simulink model "CNN_CA_control_six_springs"  (R2024b)
settings: Solver=VariableStepAuto  StartTime=0.0  StopTime=30  RelTol=1e-3
model workspace (MAT data in the model file):
  Camera1 = 1
undefined symbols (not defined in the file or in its folder): arm_radius, control_section_number, floor_radius, ini_arm_length, ini_spring_length, section_thickness, spring_position_scale, spring_radius, spring_stiffness, X, Y, Z
libraries: sm_lib x304, nesl_utility x156, dspindex x60, deeplib x1
(part 1 of 12)
settings Model: SimulationMode=accelerator  Creator=Fan Ye  LastModifiedBy=elija
settings SolverCC: AlgebraicLoopSolver=TrustRegion
settings OptimizationCC: ReuseModelBlockBuffer=off
settings DebuggingCC: UnconnectedInputMsg=warning  UnconnectedOutputMsg=warning  UnconnectedLineMsg=warning
settings ModelReferenceCC: EnableRefExpFcnMdlSchedulingChecks=on
settings SFSimCC: SimGenImportedTypeDefs=on  SimTargetLang=C++
settings RTWCC: GPUComputeCapability=3.5  DLArmComputeVersion=19.05
settings ExplorerConfigSet: InternalSimMechanicsExplorerSettings="<ExplorerConfiguration><canonicalview>default</canonicalview><AnimationSetting><BasePlaybackSpeed>1.0</BasePlaybackSpeed><PlaybackSpeedFactor>1.0</PlaybackSpeedFactor></AnimationSetting><TilePanel><TileInfo><Tiles Columns=\"1\" Count=\"1\" Rows=\"1\"><Column Weight=\"1\"/><Row Weight=\"1\"/><Tile Height=\"1\" Width=\"1\" X=\"0\" Y=\"0\"/></Tiles></TileInfo><SceneInfo><SceneViewer><BGColor><R>0.60000002384185791</R><G>0.60000002384185791</G><B>0.60000002384185791</B></BGColor><Camera><DoPerspective>off</DoPerspective><Position><X>0.561995715374629667</X><Y>-0.564875895152751606</Y><Z>0.957601428231976137</Z></Position><Center><X>-0.0153545538149960289</X><Y>0.0124743740368741876</Y><Z>0.380251159042350184</Z></Center><Up><X>-0.408248290463863073</X><Y>0.408248290463863073</Y><Z>0.816496580927726145</Z></Up><ViewLimDist>1</ViewLimDist><YLim>0.539098595499992506</YLim><XLim>0.631280340074036994</XLim></Camera></SceneViewer></SceneInfo></TilePanel><MechEditorPanel><Cameras/><GfxPanelCameraMap/><VideoCreator><PlaybackSpeedRatio>1.0</PlaybackSpeedRatio><FrameRate>1</FrameRate><VideoFormat>Motion JPEG AVI</VideoFormat><FrameSize>auto</FrameSize></VideoCreator></MechEditorPanel></ExplorerConfiguration>"

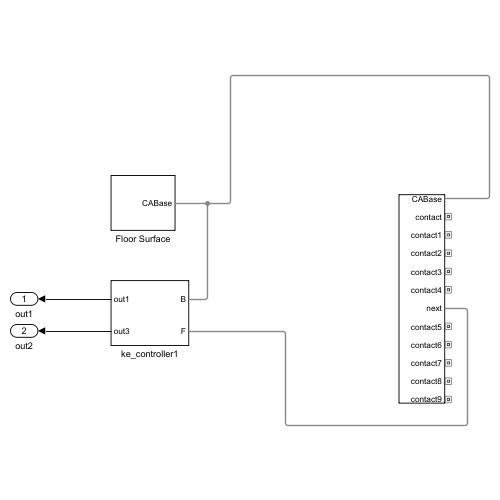
[thumbnail: Simulink's stored preview of the top-level diagram]
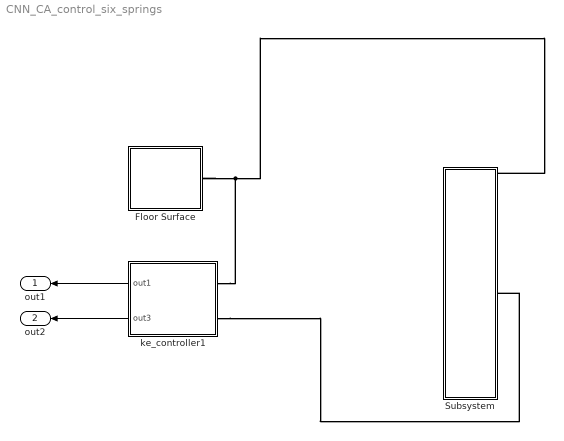
== system CNN_CA_control_six_springs ==
  Floor Surface : Subsystem  mask{length=0.5, width=0.5, floor_radius=floor_radius, floor_thickness=section_thickness, floor_density=1000}
      mask prompts: length "grid length [m]"; width "grid width [m]"; floor_radius "floor radius [m]"; floor_thickness "floor thickness [m]"; floor_density "floor density [kg/m^3]"
  Subsystem : Subsystem  mask{damping=10000}
  ke_controller1 : Subsystem  mask{time=1/10}
      settings: PortSchema="{\"entries\":[{\"content\":{\"sides\":[{\"content\":{\"connectorIds\":[\"Out1\",\"Out2\"]},\"type\":\"ConnectorPlacement.EquallySpacedRectSide\",\"uuid\":\"040155ee-60b1-421c-8328-c25461da302b\"},{\"content\":{\"connectorIds\":[\"RConn1\",\"RConn2\"],\"side\":\"RIGHT\"},\"type\":\"ConnectorPlacement.EquallySpacedRectSide\",\"uuid\":\"fd708fec-fd39-4a33-8156-5c69a86363e4\"},{\"content\":{\"connectorIds\":[],\"side\":\"TOP\"},\"type\":\"ConnectorPlacement.EquallySpacedRectSide\",\"uuid\":\"3eab7f87-5dcc-46aa-aa6d-ebff8fc02a1f\"},{\"content\":{\"connectorIds\":[],\"side\":\"HIDDEN\"},\"type\":\"ConnectorPlacement.EquallySpacedRectSide\",\"uuid\":\"eabd9a25-303c-4f3d-a71b-72a20e95be15\"}]},\"type\":\"ConnectorPlacement.EquallySpacedConnector\",\"uuid\":\"7f057b11-92ee-4c15-b9f6-e9a247ee9eef\"}],\"packageUris\":[\"http://schema.mathworks.com/mf0/Connector/R2020b\"],\"version\":\"1.0\"}"
  out1 : Outport
  out2 : Outport  Port=2
  wires:
  ke_controller1/1(out1) -> out1/1
  ke_controller1/2(out3) -> out2/1
  connections:
  Floor Surface/RConn1 -- ke_controller1/RConn1 -- Subsystem/RConn1
  ke_controller1/RConn2 -- Subsystem/RConn7

== system CNN_CA_control_six_springs/Floor Surface ==
  Floor : Subsystem  AncestorBlock=RP_Simulator_Components/Obstacle Arena/Floor
      settings: LibrarySourceBlock=RP_Simulator_Components/Obstacle Arena/Floor
  Mechanism Configuration1 : sm_lib/Utilities/Mechanism Configuration  UniformGravity=Constant  GravityVector=[0 0 9.80665]  GravityVectorUnits=m/s^2  LinearizationDelta=0.001  JointModeTransitionNonlinearIterations=2
  Solver Configuration1 : nesl_utility/Solver Configuration  PhysicalDomain=network_engine_domain  SubClassName=solver  LeftPortType=input  RightPortType=generic  Tones=[]  Harmonics=[]  SimulateNoise=off  Profile=off  UseLocalSampling=off  EnableSwitchedLinearOptims=on  FrequencyDomain=off  UseCCode=off  RelTol=0.001  AbsTol=1e-06  MinStep=1e-09  ToWorkspace=off  RevertToSquareIcSolve=off  NumHomotopyIterations=100  PhasorMode=off  PhasorModeNumHarmonics=1  ConsistencySolver=NEWTON_FTOL  IndexReductionMethod=DerivativeReplacement  DoDC=off  ResidualTolerance=1e-09  ConsistencyTolSource=GLOBAL  ConsistencyAbsTol=0.001  ConsistencyRelTol=0.001  ConsistencyTolFactor=0.001  UseLocalSolver=off  LocalSolverChoice=NE_BACKWARD_EULER_ADVANCER  ResolveIndetEquations=on  FunctionEvalNumThread=1  LocalSolverSampleTime=0.0002  DoFixedCost=off  MaxNonlinIter=10  MaxModeIter=2  ComputeImpulses=off  ImpulseIterations=2  LinearAlgebra=Sparse  LinearAlgebraNumThread=0  EquationFormulation=NE_TIME_EF  DelaysMemoryBudget=1024  AutomaticFiltering=off  FilteringTimeConstant=0.001  PartitionStorageMethod=AS_NEEDED  PartitionMemoryBudget=1024  PartitionMethod=FAST  MultibodyUseLocalSolver=off  MultibodyLocalSolverChoice=ODE1  MultibodyLocalSolverSampleTime=0.001
  World Frame1 : sm_lib/Frames and Transforms/World Frame
  CABase : PMIOPort  Side=Right
  connections:
  Floor/RConn1 -- CABase/RConn1 -- Mechanism Configuration1/RConn1 -- World Frame1/RConn1 -- Solver Configuration1/RConn1

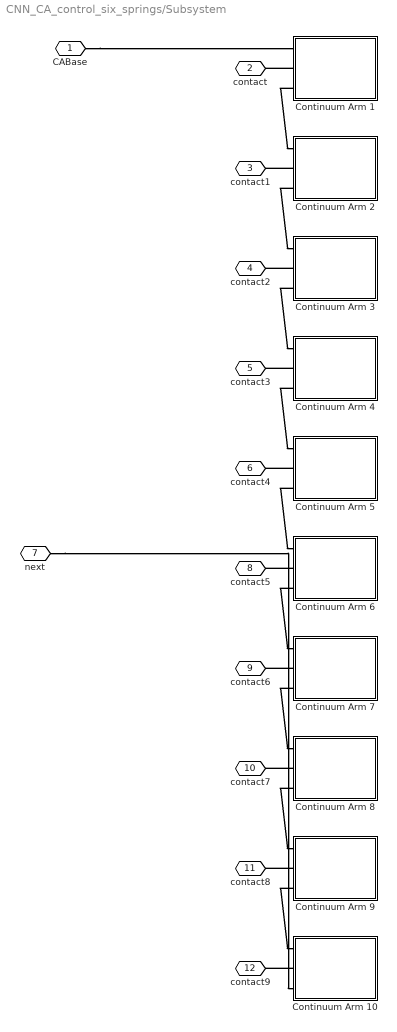
== system CNN_CA_control_six_springs/Subsystem ==
  Continuum Arm 1 : Subsystem  mask{arm_radius=arm_radius(1), arm_radius_previus=floor_radius, arm_thickness=section_thickness, arm_mass=0.00001, spring_radius=spring_radius(1), spring_mass=0.00001, ini_arm_length=ini_arm_length(1), column_number=control_section_number(1), spring_position_scale_1=spring_position_scale(1,1), spring_stiffness_1=spring_stiffness(1,1), damping_coefficient_1=damping, ini_spring_length_1=ini_spring_length(1,1), spring_position_scale_2=spring_position_scale(1,2), spring_stiffness_2=spring_stiffness(1,2), damping_coefficient_2=damping, ini_spring_length_2=ini_spring_length(1,2), spring_position_scale_3=spring_position_scale(1,3), spring_stiffness_3=spring_stiffness(1,3), damping_coefficient_3=damping, ini_spring_length_3=ini_spring_length(1,3)}
      mask prompts: arm_radius "arm radius [m]"; arm_radius_previus "arm radius previus [m]"; arm_thickness "arm thickness [m]"; arm_mass "arm mass [kg]"; spring_radius "spring radius [m]"; spring_mass "spring mass [kg]"; ini_arm_length "ini arm length [m]"; column_number "control section number"; spring_position_scale_1 "spring position scale"; spring_stiffness_1 "spring stiffness [N/m]"; damping_coefficient_1 "damping coefficient [N/(m/s)]"; ini_spring_length_1 "ini spring length [m]"; spring_position_scale_2 "spring position scale"; spring_stiffness_2 "spring stiffness [N/m]"; damping_coefficient_2 "damping coefficient [N/(m/s)]"; ini_spring_length_2 "ini spring length [m]"; spring_position_scale_3 "spring position scale"; spring_stiffness_3 "spring stiffness [N/m]"; damping_coefficient_3 "damping coefficient [N/(m/s)]"; ini_spring_length_3 "ini spring length [m]"
      mask DialogControl spring1 Prompt: spring1
      mask DialogControl spring2 Prompt: spring2
      mask DialogControl spring3 Prompt: spring3
  Continuum Arm 10 : Subsystem  mask{arm_radius=arm_radius(10), arm_radius_previus=arm_radius(9), arm_thickness=section_thickness, arm_mass=0.00001, spring_radius=spring_radius(10), spring_mass=0.00001, ini_arm_length=ini_arm_length(10), column_number=control_section_number(10), spring_position_scale_1=spring_position_scale(10,1), spring_stiffness_1=spring_stiffness(10,1), damping_coefficient_1=damping, ini_spring_length_1=ini_spring_length(10,1), spring_position_scale_2=spring_position_scale(10,2), spring_stiffness_2=spring_stiffness(10,2), damping_coefficient_2=damping, ini_spring_length_2=ini_spring_length(10,2), spring_position_scale_3=spring_position_scale(10,3), spring_stiffness_3=spring_stiffness(10,3), damping_coefficient_3=damping, ini_spring_length_3=ini_spring_length(10,3)}
      mask prompts: arm_radius "arm radius [m]"; arm_radius_previus "arm radius previus [m]"; arm_thickness "arm thickness [m]"; arm_mass "arm mass [kg]"; spring_radius "spring radius [m]"; spring_mass "spring mass [kg]"; ini_arm_length "ini arm length [m]"; column_number "control section number"; spring_position_scale_1 "spring position scale"; spring_stiffness_1 "spring stiffness [N/m]"; damping_coefficient_1 "damping coefficient [N/(m/s)]"; ini_spring_length_1 "ini spring length [m]"; spring_position_scale_2 "spring position scale"; spring_stiffness_2 "spring stiffness [N/m]"; damping_coefficient_2 "damping coefficient [N/(m/s)]"; ini_spring_length_2 "ini spring length [m]"; spring_position_scale_3 "spring position scale"; spring_stiffness_3 "spring stiffness [N/m]"; damping_coefficient_3 "damping coefficient [N/(m/s)]"; ini_spring_length_3 "ini spring length [m]"
      mask DialogControl spring1 Prompt: spring1
      mask DialogControl spring2 Prompt: spring2
      mask DialogControl spring3 Prompt: spring3
  Continuum Arm 2 : Subsystem  mask{arm_radius=arm_radius(2), arm_radius_previus=arm_radius(1), arm_thickness=section_thickness, arm_mass=0.00001, spring_radius=spring_radius(2), spring_mass=0.00001, ini_arm_length=ini_arm_length(2), column_number=control_section_number(2), spring_position_scale_1=spring_position_scale(2,1), spring_stiffness_1=spring_stiffness(2,1), damping_coefficient_1=damping, ini_spring_length_1=ini_spring_length(2,1), spring_position_scale_2=spring_position_scale(2,2), spring_stiffness_2=spring_stiffness(2,2), damping_coefficient_2=damping, ini_spring_length_2=ini_spring_length(2,2), spring_position_scale_3=spring_position_scale(2,3), spring_stiffness_3=spring_stiffness(2,3), damping_coefficient_3=damping, ini_spring_length_3=ini_spring_length(2,3)}
      mask prompts: arm_radius "arm radius [m]"; arm_radius_previus "arm radius previus [m]"; arm_thickness "arm thickness [m]"; arm_mass "arm mass [kg]"; spring_radius "spring radius [m]"; spring_mass "spring mass [kg]"; ini_arm_length "ini arm length [m]"; column_number "control section number"; spring_position_scale_1 "spring position scale"; spring_stiffness_1 "spring stiffness [N/m]"; damping_coefficient_1 "damping coefficient [N/(m/s)]"; ini_spring_length_1 "ini spring length [m]"; spring_position_scale_2 "spring position scale"; spring_stiffness_2 "spring stiffness [N/m]"; damping_coefficient_2 "damping coefficient [N/(m/s)]"; ini_spring_length_2 "ini spring length [m]"; spring_position_scale_3 "spring position scale"; spring_stiffness_3 "spring stiffness [N/m]"; damping_coefficient_3 "damping coefficient [N/(m/s)]"; ini_spring_length_3 "ini spring length [m]"
      mask DialogControl spring1 Prompt: spring1
      mask DialogControl spring2 Prompt: spring2
      mask DialogControl spring3 Prompt: spring3
  Continuum Arm 3 : Subsystem  mask{arm_radius=arm_radius(3), arm_radius_previus=arm_radius(2), arm_thickness=section_thickness, arm_mass=0.00001, spring_radius=spring_radius(3), spring_mass=0.00001, ini_arm_length=ini_arm_length(3), column_number=control_section_number(3), spring_position_scale_1=spring_position_scale(3,1), spring_stiffness_1=spring_stiffness(3,1), damping_coefficient_1=damping, ini_spring_length_1=ini_spring_length(3,1), spring_position_scale_2=spring_position_scale(3,2), spring_stiffness_2=spring_stiffness(3,2), damping_coefficient_2=damping, ini_spring_length_2=ini_spring_length(3,2), spring_position_scale_3=spring_position_scale(3,3), spring_stiffness_3=spring_stiffness(3,3), damping_coefficient_3=damping, ini_spring_length_3=ini_spring_length(3,3)}
      mask prompts: arm_radius "arm radius [m]"; arm_radius_previus "arm radius previus [m]"; arm_thickness "arm thickness [m]"; arm_mass "arm mass [kg]"; spring_radius "spring radius [m]"; spring_mass "spring mass [kg]"; ini_arm_length "ini arm length [m]"; column_number "control section number"; spring_position_scale_1 "spring position scale"; spring_stiffness_1 "spring stiffness [N/m]"; damping_coefficient_1 "damping coefficient [N/(m/s)]"; ini_spring_length_1 "ini spring length [m]"; spring_position_scale_2 "spring position scale"; spring_stiffness_2 "spring stiffness [N/m]"; damping_coefficient_2 "damping coefficient [N/(m/s)]"; ini_spring_length_2 "ini spring length [m]"; spring_position_scale_3 "spring position scale"; spring_stiffness_3 "spring stiffness [N/m]"; damping_coefficient_3 "damping coefficient [N/(m/s)]"; ini_spring_length_3 "ini spring length [m]"
      mask DialogControl spring1 Prompt: spring1
      mask DialogControl spring2 Prompt: spring2
      mask DialogControl spring3 Prompt: spring3
  Continuum Arm 4 : Subsystem  mask{arm_radius=arm_radius(4), arm_radius_previus=arm_radius(3), arm_thickness=section_thickness, arm_mass=0.00001, spring_radius=spring_radius(4), spring_mass=0.00001, ini_arm_length=ini_arm_length(4), column_number=control_section_number(4), spring_position_scale_1=spring_position_scale(4,1), spring_stiffness_1=spring_stiffness(4,1), damping_coefficient_1=damping, ini_spring_length_1=ini_spring_length(4,1), spring_position_scale_2=spring_position_scale(4,2), spring_stiffness_2=spring_stiffness(4,2), damping_coefficient_2=damping, ini_spring_length_2=ini_spring_length(4,2), spring_position_scale_3=spring_position_scale(4,3), spring_stiffness_3=spring_stiffness(4,3), damping_coefficient_3=damping, ini_spring_length_3=ini_spring_length(4,3)}
      mask prompts: arm_radius "arm radius [m]"; arm_radius_previus "arm radius previus [m]"; arm_thickness "arm thickness [m]"; arm_mass "arm mass [kg]"; spring_radius "spring radius [m]"; spring_mass "spring mass [kg]"; ini_arm_length "ini arm length [m]"; column_number "control section number"; spring_position_scale_1 "spring position scale"; spring_stiffness_1 "spring stiffness [N/m]"; damping_coefficient_1 "damping coefficient [N/(m/s)]"; ini_spring_length_1 "ini spring length [m]"; spring_position_scale_2 "spring position scale"; spring_stiffness_2 "spring stiffness [N/m]"; damping_coefficient_2 "damping coefficient [N/(m/s)]"; ini_spring_length_2 "ini spring length [m]"; spring_position_scale_3 "spring position scale"; spring_stiffness_3 "spring stiffness [N/m]"; damping_coefficient_3 "damping coefficient [N/(m/s)]"; ini_spring_length_3 "ini spring length [m]"
      mask DialogControl spring1 Prompt: spring1
      mask DialogControl spring2 Prompt: spring2
      mask DialogControl spring3 Prompt: spring3
  Continuum Arm 5 : Subsystem  mask{arm_radius=arm_radius(5), arm_radius_previus=arm_radius(4), arm_thickness=section_thickness, arm_mass=0.00001, spring_radius=spring_radius(5), spring_mass=0.00001, ini_arm_length=ini_arm_length(5), column_number=control_section_number(5), spring_position_scale_1=spring_position_scale(5,1), spring_stiffness_1=spring_stiffness(5,1), damping_coefficient_1=damping, ini_spring_length_1=ini_spring_length(5,1), spring_position_scale_2=spring_position_scale(5,2), spring_stiffness_2=spring_stiffness(5,2), damping_coefficient_2=damping, ini_spring_length_2=ini_spring_length(5,2), spring_position_scale_3=spring_position_scale(5,3), spring_stiffness_3=spring_stiffness(5,3), damping_coefficient_3=damping, ini_spring_length_3=ini_spring_length(5,3)}
      mask prompts: arm_radius "arm radius [m]"; arm_radius_previus "arm radius previus [m]"; arm_thickness "arm thickness [m]"; arm_mass "arm mass [kg]"; spring_radius "spring radius [m]"; spring_mass "spring mass [kg]"; ini_arm_length "ini arm length [m]"; column_number "control section number"; spring_position_scale_1 "spring position scale"; spring_stiffness_1 "spring stiffness [N/m]"; damping_coefficient_1 "damping coefficient [N/(m/s)]"; ini_spring_length_1 "ini spring length [m]"; spring_position_scale_2 "spring position scale"; spring_stiffness_2 "spring stiffness [N/m]"; damping_coefficient_2 "damping coefficient [N/(m/s)]"; ini_spring_length_2 "ini spring length [m]"; spring_position_scale_3 "spring position scale"; spring_stiffness_3 "spring stiffness [N/m]"; damping_coefficient_3 "damping coefficient [N/(m/s)]"; ini_spring_length_3 "ini spring length [m]"
      mask DialogControl spring1 Prompt: spring1
      mask DialogControl spring2 Prompt: spring2
      mask DialogControl spring3 Prompt: spring3
  Continuum Arm 6 : Subsystem  mask{arm_radius=arm_radius(6), arm_radius_previus=arm_radius(5), arm_thickness=section_thickness, arm_mass=0.00001, spring_radius=spring_radius(6), spring_mass=0.00001, ini_arm_length=ini_arm_length(6), column_number=control_section_number(6), spring_position_scale_1=spring_position_scale(6,1), spring_stiffness_1=spring_stiffness(6,1), damping_coefficient_1=damping, ini_spring_length_1=ini_spring_length(6,1), spring_position_scale_2=spring_position_scale(6,2), spring_stiffness_2=spring_stiffness(6,2), damping_coefficient_2=damping, ini_spring_length_2=ini_spring_length(6,2), spring_position_scale_3=spring_position_scale(6,3), spring_stiffness_3=spring_stiffness(6,3), damping_coefficient_3=damping, ini_spring_length_3=ini_spring_length(6,3)}
      mask prompts: arm_radius "arm radius [m]"; arm_radius_previus "arm radius previus [m]"; arm_thickness "arm thickness [m]"; arm_mass "arm mass [kg]"; spring_radius "spring radius [m]"; spring_mass "spring mass [kg]"; ini_arm_length "ini arm length [m]"; column_number "control section number"; spring_position_scale_1 "spring position scale"; spring_stiffness_1 "spring stiffness [N/m]"; damping_coefficient_1 "damping coefficient [N/(m/s)]"; ini_spring_length_1 "ini spring length [m]"; spring_position_scale_2 "spring position scale"; spring_stiffness_2 "spring stiffness [N/m]"; damping_coefficient_2 "damping coefficient [N/(m/s)]"; ini_spring_length_2 "ini spring length [m]"; spring_position_scale_3 "spring position scale"; spring_stiffness_3 "spring stiffness [N/m]"; damping_coefficient_3 "damping coefficient [N/(m/s)]"; ini_spring_length_3 "ini spring length [m]"
      mask DialogControl spring1 Prompt: spring1
      mask DialogControl spring2 Prompt: spring2
      mask DialogControl spring3 Prompt: spring3
  Continuum Arm 7 : Subsystem  mask{arm_radius=arm_radius(7), arm_radius_previus=arm_radius(6), arm_thickness=section_thickness, arm_mass=0.00001, spring_radius=spring_radius(7), spring_mass=0.00001, ini_arm_length=ini_arm_length(7), column_number=control_section_number(7), spring_position_scale_1=spring_position_scale(7,1), spring_stiffness_1=spring_stiffness(7,1), damping_coefficient_1=damping, ini_spring_length_1=ini_spring_length(7,1), spring_position_scale_2=spring_position_scale(7,2), spring_stiffness_2=spring_stiffness(7,2), damping_coefficient_2=damping, ini_spring_length_2=ini_spring_length(7,2), spring_position_scale_3=spring_position_scale(7,3), spring_stiffness_3=spring_stiffness(7,3), damping_coefficient_3=damping, ini_spring_length_3=ini_spring_length(7,3)}
      mask prompts: arm_radius "arm radius [m]"; arm_radius_previus "arm radius previus [m]"; arm_thickness "arm thickness [m]"; arm_mass "arm mass [kg]"; spring_radius "spring radius [m]"; spring_mass "spring mass [kg]"; ini_arm_length "ini arm length [m]"; column_number "control section number"; spring_position_scale_1 "spring position scale"; spring_stiffness_1 "spring stiffness [N/m]"; damping_coefficient_1 "damping coefficient [N/(m/s)]"; ini_spring_length_1 "ini spring length [m]"; spring_position_scale_2 "spring position scale"; spring_stiffness_2 "spring stiffness [N/m]"; damping_coefficient_2 "damping coefficient [N/(m/s)]"; ini_spring_length_2 "ini spring length [m]"; spring_position_scale_3 "spring position scale"; spring_stiffness_3 "spring stiffness [N/m]"; damping_coefficient_3 "damping coefficient [N/(m/s)]"; ini_spring_length_3 "ini spring length [m]"
      mask DialogControl spring1 Prompt: spring1
      mask DialogControl spring2 Prompt: spring2
      mask DialogControl spring3 Prompt: spring3
  Continuum Arm 8 : Subsystem  mask{arm_radius=arm_radius(8), arm_radius_previus=arm_radius(7), arm_thickness=section_thickness, arm_mass=0.00001, spring_radius=spring_radius(8), spring_mass=0.00001, ini_arm_length=ini_arm_length(8), column_number=control_section_number(8), spring_position_scale_1=spring_position_scale(8,1), spring_stiffness_1=spring_stiffness(8,1), damping_coefficient_1=damping, ini_spring_length_1=ini_spring_length(8,1), spring_position_scale_2=spring_position_scale(8,2), spring_stiffness_2=spring_stiffness(8,2), damping_coefficient_2=damping, ini_spring_length_2=ini_spring_length(8,2), spring_position_scale_3=spring_position_scale(8,3), spring_stiffness_3=spring_stiffness(8,3), damping_coefficient_3=damping, ini_spring_length_3=ini_spring_length(8,3)}
      mask prompts: arm_radius "arm radius [m]"; arm_radius_previus "arm radius previus [m]"; arm_thickness "arm thickness [m]"; arm_mass "arm mass [kg]"; spring_radius "spring radius [m]"; spring_mass "spring mass [kg]"; ini_arm_length "ini arm length [m]"; column_number "control section number"; spring_position_scale_1 "spring position scale"; spring_stiffness_1 "spring stiffness [N/m]"; damping_coefficient_1 "damping coefficient [N/(m/s)]"; ini_spring_length_1 "ini spring length [m]"; spring_position_scale_2 "spring position scale"; spring_stiffness_2 "spring stiffness [N/m]"; damping_coefficient_2 "damping coefficient [N/(m/s)]"; ini_spring_length_2 "ini spring length [m]"; spring_position_scale_3 "spring position scale"; spring_stiffness_3 "spring stiffness [N/m]"; damping_coefficient_3 "damping coefficient [N/(m/s)]"; ini_spring_length_3 "ini spring length [m]"
      mask DialogControl spring1 Prompt: spring1
      mask DialogControl spring2 Prompt: spring2
      mask DialogControl spring3 Prompt: spring3
  Continuum Arm 9 : Subsystem  mask{arm_radius=arm_radius(9), arm_radius_previus=arm_radius(8), arm_thickness=section_thickness, arm_mass=0.00001, spring_radius=spring_radius(9), spring_mass=0.00001, ini_arm_length=ini_arm_length(9), column_number=control_section_number(9), spring_position_scale_1=spring_position_scale(9,1), spring_stiffness_1=spring_stiffness(9,1), damping_coefficient_1=damping, ini_spring_length_1=ini_spring_length(9,1), spring_position_scale_2=spring_position_scale(9,2), spring_stiffness_2=spring_stiffness(9,2), damping_coefficient_2=damping, ini_spring_length_2=ini_spring_length(9,2), spring_position_scale_3=spring_position_scale(9,3), spring_stiffness_3=spring_stiffness(9,3), damping_coefficient_3=damping, ini_spring_length_3=ini_spring_length(9,3)}
      mask prompts: arm_radius "arm radius [m]"; arm_radius_previus "arm radius previus [m]"; arm_thickness "arm thickness [m]"; arm_mass "arm mass [kg]"; spring_radius "spring radius [m]"; spring_mass "spring mass [kg]"; ini_arm_length "ini arm length [m]"; column_number "control section number"; spring_position_scale_1 "spring position scale"; spring_stiffness_1 "spring stiffness [N/m]"; damping_coefficient_1 "damping coefficient [N/(m/s)]"; ini_spring_length_1 "ini spring length [m]"; spring_position_scale_2 "spring position scale"; spring_stiffness_2 "spring stiffness [N/m]"; damping_coefficient_2 "damping coefficient [N/(m/s)]"; ini_spring_length_2 "ini spring length [m]"; spring_position_scale_3 "spring position scale"; spring_stiffness_3 "spring stiffness [N/m]"; damping_coefficient_3 "damping coefficient [N/(m/s)]"; ini_spring_length_3 "ini spring length [m]"
      mask DialogControl spring1 Prompt: spring1
      mask DialogControl spring2 Prompt: spring2
      mask DialogControl spring3 Prompt: spring3
  CABase : PMIOPort  Side=Right
  contact : PMIOPort  Port=2  Side=Right
  contact1 : PMIOPort  Port=3  Side=Right
  contact2 : PMIOPort  Port=4  Side=Right
  contact3 : PMIOPort  Port=5  Side=Right
  contact4 : PMIOPort  Port=6  Side=Right
  next : PMIOPort  Port=7  Side=Right
  contact5 : PMIOPort  Port=8  Side=Right
  contact6 : PMIOPort  Port=9  Side=Right
  contact7 : PMIOPort  Port=10  Side=Right
  contact8 : PMIOPort  Port=11  Side=Right
  contact9 : PMIOPort  Port=12  Side=Right
  connections:
  Continuum Arm 1/RConn3 -- Continuum Arm 2/RConn1
  Continuum Arm 3/RConn3 -- Continuum Arm 4/RConn1
  Continuum Arm 7/RConn3 -- Continuum Arm 8/RConn1
  Continuum Arm 2/RConn2 -- contact1/RConn1
  Continuum Arm 8/RConn3 -- Continuum Arm 9/RConn1
  Continuum Arm 2/RConn3 -- Continuum Arm 3/RConn1
  Continuum Arm 6/RConn3 -- Continuum Arm 7/RConn1
  Continuum Arm 3/RConn2 -- contact2/RConn1
  Continuum Arm 5/RConn3 -- Continuum Arm 6/RConn1
  Continuum Arm 9/RConn3 -- Continuum Arm 10/RConn1
  Continuum Arm 4/RConn3 -- Continuum Arm 5/RConn1
  next/RConn1 -- Continuum Arm 10/RConn3
  CABase/RConn1 -- Continuum Arm 1/RConn1
  Continuum Arm 5/RConn2 -- contact4/RConn1
  Continuum Arm 1/RConn2 -- contact/RConn1
  Continuum Arm 9/RConn2 -- contact8/RConn1
  Continuum Arm 10/RConn2 -- contact9/RConn1
  Continuum Arm 7/RConn2 -- contact6/RConn1
  Continuum Arm 8/RConn2 -- contact7/RConn1
  Continuum Arm 4/RConn2 -- contact3/RConn1
  Continuum Arm 6/RConn2 -- contact5/RConn1

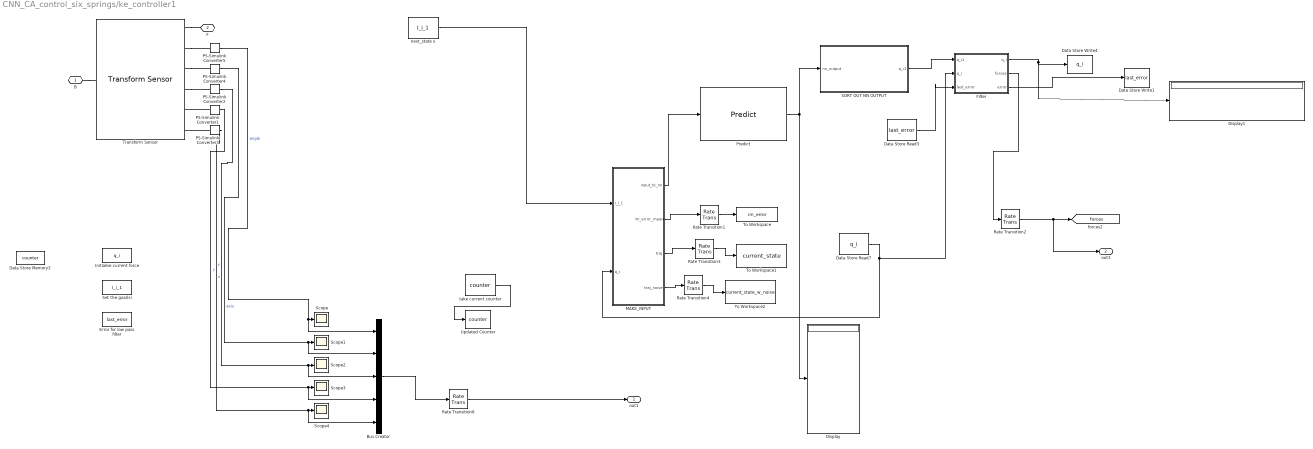
== system CNN_CA_control_six_springs/ke_controller1 ==
  Bus Creator : BusCreator  Inputs=5
  Data Store Memory3 : DataStoreMemory  DataStoreName=counter  WriteAfterWriteMsg=warning  InitialValue=counter  ShowAdditionalParam=off
  Data Store Read3 : DataStoreRead  DataStoreName=last_error  IndexOptions=Index vector (dialog)  Indices=1  OutputSizes=1
  Data Store Read7 : DataStoreRead  DataStoreName=q_i  IndexOptions=Index vector (dialog)  Indices=1  OutputSizes=1
  Data Store Write1 : DataStoreWrite  DataStoreName=last_error  IndexOptions=Index vector (dialog)  Indices=1  OutputSizes=1
  Data Store Write4 : DataStoreWrite  DataStoreName=q_i  IndexOptions=Index vector (dialog)  Indices=1  OutputSizes=1
  Display : Display
  Display1 : Display
  Error for low pass filter : DataStoreMemory  DataStoreName=last_error  WriteAfterWriteMsg=warning  InitialValue=last_error  ShowAdditionalParam=off
  Filter : MATLAB Function  TreatAsAtomicUnit=on  SystemSampleTime=time
  Initialise current force : DataStoreMemory  DataStoreName=q_i  WriteAfterWriteMsg=warning  InitialValue=q_i  ShowAdditionalParam=off
  MAKE_INPUT : MATLAB Function  TreatAsAtomicUnit=on  SystemSampleTime=time
  PS-Simulink Converter{1..5} (5 alike) : nesl_utility/PS-Simulink Converter  PhysicalDomain=network_engine_domain  SubClassName=ps_output  LeftPortType=input  RightPortType=output  PseudoPeriodic=off  Frequencies=[]  VectorFormat=1-D array  Unit=1  AffineConversion=off
  Predict : deeplib/Predict  Network=Network from MAT-file  NetworkFunction=squeezenet  NetworkFilePath=.\variable_net6_best.mat  MiniBatchSize=1  InputDataFormats={'',''}  Predictions=on  Activations={}  ForceInterpretedSim=off  EnableDLNetwork=on  LastKnownNetworkFilePath=''  LastKnownNetworkTimeStamp=''
  Rate Transition{1..4,8} (5 alike) : RateTransition  OutPortSampleTime=time
  SORT OUT NN OUTPUT : MATLAB Function  TreatAsAtomicUnit=on  SystemSampleTime=0.1
  Scope{,1..4} (5 alike) : Scope
  Set the goal(s) : DataStoreMemory  DataStoreName=I_i_1  WriteAfterWriteMsg=warning  InitialValue=I_i_1  ShowAdditionalParam=off
  To Workspace : ToWorkspace  VariableName=im_error  SaveFormat=Timeseries  SampleTime=-1
  To Workspace1 : ToWorkspace  VariableName=current_state  SaveFormat=Timeseries  SampleTime=-1
  To Workspace2 : ToWorkspace  VariableName=current_state_w_noise  SaveFormat=Timeseries  SampleTime=-1
  Transform Sensor : sm_lib/Frames and Transforms/Transform Sensor  MeasurementFrame=World  RotationSequence=XYX  SenseAngle=on  SenseAxis=on  SenseQ=off  SenseR=off  SenseRotationSequence=off  SenseOmegaX=off  SenseOmegaY=off  SenseOmegaZ=off  SenseOmega=off  SenseQDot=off  SenseRDot=off  SenseRotationSequenceDot=off  SenseAlphaX=off  SenseAlphaY=off  SenseAlphaZ=off  SenseAlpha=off  SenseQDDot=off  SenseRDDot=off  SenseX=on  SenseY=on  SenseZ=on  SenseXYZ=off  SenseRad=off  SenseAzim=off  SenseDist=off  SenseInc=off  SenseXDot=off  SenseYDot=off  SenseZDot=off  SenseXYZDot=off  SenseRadDot=off  SenseAzimDot=off  SenseDistDot=off  SenseIncDot=off  SenseXDDot=off  SenseYDDot=off  SenseZDDot=off  SenseXYZDDot=off  SenseRadDDot=off  SenseAzimDDot=off  SenseDistDDot=off  SenseIncDDot=off
  Updated Counter : DataStoreWrite  DataStoreName=counter  IndexOptions=Index vector (dialog)  Indices=1  OutputSizes=1
  next_state x : DataStoreRead  DataStoreName=I_i_1  IndexOptions=Index vector (dialog)  Indices=1  OutputSizes=1
  take current counter : DataStoreRead  DataStoreName=counter  IndexOptions=Index vector (dialog)  Indices=1  OutputSizes=1
  B : PMIOPort  Side=Right
  F : PMIOPort  Port=2  Side=Right
  out1 : Outport
  out3 : Outport  Port=2
  tag scope: forces=global
  wires:
  PS-Simulink Converter3/1 -> Bus Creator/5, Scope4/1  "z"
  PS-Simulink Converter1/1 -> Bus Creator/4, Scope3/1  "y"
  PS-Simulink Converter2/1 -> Bus Creator/3, Scope2/1  "x"
  PS-Simulink Converter4/1 -> Bus Creator/2, Scope1/1  "axis"
  PS-Simulink Converter5/1 -> Bus Creator/1, Scope/1  "angle"
  Bus Creator/1 -> Rate Transition8/1
  Rate Transition8/1 -> out1/1
  take current counter/1 -> Updated Counter/1
  MAKE_INPUT/1(input_to_nn) -> Predict/1
  Predict/1 -> Display/1, SORT OUT NN OUTPUT/1(nn_output)
  SORT OUT NN OUTPUT/1(q_i1) -> Filter/1(q_i1)
  next_state x/1 -> MAKE_INPUT/1(I_i_1)
  Data Store Read7/1 -> Filter/2("q_i "), MAKE_INPUT/2(q_i)
  Filter/1(q_i) -> Display1/1, Data Store Write4/1
  Rate Transition2/1 -> out3/1, [forces]
  Filter/2(forces) -> Rate Transition2/1
  Data Store Read3/1 -> Filter/3(last_error)
  Filter/3(error) -> Data Store Write1/1
  MAKE_INPUT/2(im_error_mean) -> Rate Transition1/1
  Rate Transition1/1 -> To Workspace/1
  MAKE_INPUT/3(traj) -> Rate Transition3/1
  Rate Transition3/1 -> To Workspace1/1
  Rate Transition4/1 -> To Workspace2/1
  MAKE_INPUT/4(traj_noise) -> Rate Transition4/1
  connections:
  PS-Simulink Converter3/LConn1 -- Transform Sensor/RConn6
  PS-Simulink Converter1/LConn1 -- Transform Sensor/RConn5
  Transform Sensor/RConn4 -- PS-Simulink Converter2/LConn1
  Transform Sensor/RConn3 -- PS-Simulink Converter4/LConn1
  Transform Sensor/RConn2 -- PS-Simulink Converter5/LConn1
  B/RConn1 -- Transform Sensor/LConn1
  Transform Sensor/RConn1 -- F/RConn1

== system CNN_CA_control_six_springs/Floor Surface/Floor ==
  Floor : sm_lib/Body Elements/Cylindrical Solid  CylinderRadius=floor_radius  CylinderRadiusUnits=m  CylinderLength=floor_thickness  CylinderLengthUnits=m  ExportEntireGeometry=on  InertiaType=CalculateFromGeometry  BasedOnType=Density  Density=floor_density  DensityUnits=kg/m^3  Mass=0  MassUnits=kg  CenterOfMass=[0 0 0]  CenterOfMassUnits=m  MomentsOfInertia=[1 1 1]  MomentsOfInertiaUnits=kg*m^2  ProductsOfInertia=[1 1 1]  ProductsOfInertiaUnits=kg*m^2  GraphicType=FromGeometry  MarkerShape=Sphere  MarkerSize=10  GraphicVisPropType=SimpleVisualProperties  GraphicDiffuseColor=[1.0 0 0]  GraphicOpacity=1.0  GraphicSpecularColor=[0.5 0.5 0.5 1.0]  GraphicAmbientColor=[0.15 0.15 0.15 1.0]  GraphicEmissiveColor=[0.0 0.0 0.0 1.0]  GraphicShininess=75  DoExposeReferenceFrame=on  SerializedFrames=<Frames/>
  Ref : PMIOPort  Side=Right
  connections:
  Floor/RConn1 -- Ref/RConn1

== system CNN_CA_control_six_springs/Subsystem/Continuum Arm 1 ==
  Arm Slice : sm_lib/Body Elements/Cylindrical Solid  CylinderRadius=arm_radius  CylinderRadiusUnits=m  CylinderLength=arm_thickness  CylinderLengthUnits=m  ExportEntireGeometry=on  InertiaType=CalculateFromGeometry  BasedOnType=Mass  Density=1000  DensityUnits=kg/m^3  Mass=arm_mass  MassUnits=kg  CenterOfMass=[0 0 0]  CenterOfMassUnits=m  MomentsOfInertia=[1 1 1]  MomentsOfInertiaUnits=kg*m^2  ProductsOfInertia=[1 1 1]  ProductsOfInertiaUnits=kg*m^2  GraphicType=FromGeometry  MarkerShape=Sphere  MarkerSize=10  GraphicVisPropType=SimpleVisualProperties  GraphicDiffuseColor=[1.0 0 0]  GraphicOpacity=1.0  GraphicSpecularColor=[0.5 0.5 0.5 1.0]  GraphicAmbientColor=[0.15 0.15 0.15 1.0]  GraphicEmissiveColor=[0.0 0.0 0.0 1.0]  GraphicShininess=75  DoExposeReferenceFrame=on  SerializedFrames=<Frames/>
  Prismatic Joint : sm_lib/Joints/Prismatic Joint  JointMode=Normal  CompositeWrenchDir=FollowerOnBase  CompositeWrenchFrame=BaseFrame  SenseConstraintForce=off  SenseConstraintTorque=off  SenseTotalForce=off  SenseTotalTorque=off  PositionTargetSpecify=on  PositionTargetPriority=High  PositionTargetValue=ini_arm_length  PositionTargetValueUnits=m  VelocityTargetSpecify=off  VelocityTargetPriority=High  VelocityTargetValue=0  VelocityTargetValueUnits=m/s  EquilibriumPosition=0  EquilibriumPositionUnits=m  SpringStiffness=0  SpringStiffnessUnits=N/m  DampingCoefficient=0  DampingCoefficientUnits=N/(m/s)  LowerLimitSpecify=off  LowerLimitBound=-1  LowerLimitBoundUnits=m  LowerLimitStiffness=1e6  LowerLimitStiffnessUnits=N/m  LowerLimitDamping=1e3  LowerLimitDampingUnits=N/(m/s)  LowerLimitTransitionRegionWidth=1e-4  LowerLimitTransitionRegionWidthUnits=m  UpperLimitSpecify=off  UpperLimitBound=1  UpperLimitBoundUnits=m  UpperLimitStiffness=1e6  UpperLimitStiffnessUnits=N/m  UpperLimitDamping=1e3  UpperLimitDampingUnits=N/(m/s)  UpperLimitTransitionRegionWidth=1e-4  UpperLimitTransitionRegionWidthUnits=m  TorqueActuationMode=NoTorque  MotionActuationMode=ComputedMotion  SensePosition=off  SenseVelocity=off  SenseAcceleration=off  SenseTorqueForce=off  SenseLowerLimitTorqueForce=off  SenseUpperLimitTorqueForce=off
  Spring Damper 1 : Subsystem  mask{spring_position_scale=spring_position_scale_1, spring_stiffness=spring_stiffness_1, damping_coefficient=damping_coefficient_1, theta=0, row_number=1}
      mask prompts: spring_position_scale "spring position scale"; spring_stiffness "spring stiffness [N/m]"; damping_coefficient "damping coefficient [N/(m/s)]"; theta "theta [deg]"; row_number "spring label"
  Spring Damper 2 : Subsystem  mask{spring_position_scale=spring_position_scale_2, spring_stiffness=spring_stiffness_2, damping_coefficient=damping_coefficient_2, theta=120, row_number=2}
      mask prompts: spring_position_scale "spring position scale"; spring_stiffness "spring stiffness [N/m]"; damping_coefficient "damping coefficient [N/(m/s)]"; theta "theta [deg]"; row_number "spring label"
  Spring Damper 3 : Subsystem  mask{spring_position_scale=spring_position_scale_3, spring_stiffness=spring_stiffness_3, damping_coefficient=damping_coefficient_3, theta=-120, row_number=3}
      mask prompts: spring_position_scale "spring position scale"; spring_stiffness "spring stiffness [N/m]"; damping_coefficient "damping coefficient [N/(m/s)]"; theta "theta [deg]"; row_number "spring label"
  Universal Joint : sm_lib/Joints/Universal Joint  JointMode=Normal  CompositeWrenchDir=FollowerOnBase  CompositeWrenchFrame=BaseFrame  SenseConstraintForce=off  SenseConstraintTorque=off  SenseTotalForce=off  SenseTotalTorque=off  RxPositionTargetSpecify=off  RxPositionTargetPriority=High  RxPositionTargetValue=0  RxPositionTargetValueUnits=deg  RxVelocityTargetSpecify=off  RxVelocityTargetPriority=High  RxVelocityTargetValue=0  RxVelocityTargetValueUnits=deg/s  RxEquilibriumPosition=0  RxEquilibriumPositionUnits=deg  RxSpringStiffness=0  RxSpringStiffnessUnits=N*m/deg  RxDampingCoefficient=0  RxDampingCoefficientUnits=N*m/(deg/s)  RxLowerLimitSpecify=off  RxLowerLimitBound=-90  RxLowerLimitBoundUnits=deg  RxLowerLimitStiffness=1e4  RxLowerLimitStiffnessUnits=N*m/deg  RxLowerLimitDamping=10  RxLowerLimitDampingUnits=N*m/(deg/s)  RxLowerLimitTransitionRegionWidth=0.1  RxLowerLimitTransitionRegionWidthUnits=deg  RxUpperLimitSpecify=off  RxUpperLimitBound=90  RxUpperLimitBoundUnits=deg  RxUpperLimitStiffness=1e4  RxUpperLimitStiffnessUnits=N*m/deg  RxUpperLimitDamping=10  RxUpperLimitDampingUnits=N*m/(deg/s)  RxUpperLimitTransitionRegionWidth=0.1  RxUpperLimitTransitionRegionWidthUnits=deg  RxTorqueActuationMode=NoTorque  RxMotionActuationMode=ComputedMotion  RxSensePosition=off  RxSenseVelocity=off  RxSenseAcceleration=off  RxSenseTorqueForce=off  RxSenseLowerLimitTorqueForce=off  RxSenseUpperLimitTorqueForce=off  RyPositionTargetSpecify=off  RyPositionTargetPriority=High  RyPositionTargetValue=0  RyPositionTargetValueUnits=deg  RyVelocityTargetSpecify=off  RyVelocityTargetPriority=High  RyVelocityTargetValue=0  RyVelocityTargetValueUnits=deg/s  RyEquilibriumPosition=0  RyEquilibriumPositionUnits=deg  RySpringStiffness=0  RySpringStiffnessUnits=N*m/deg  RyDampingCoefficient=0  RyDampingCoefficientUnits=N*m/(deg/s)  RyLowerLimitSpecify=off  RyLowerLimitBound=-90  RyLowerLimitBoundUnits=deg  RyLowerLimitStiffness=1e4  RyLowerLimitStiffnessUnits=N*m/deg  RyLowerLimitDamping=10  RyLowerLimitDampingUnits=N*m/(deg/s)  RyLowerLimitTransitionRegionWidth=0.1  RyLowerLimitTransitionRegionWidthUnits=deg  RyUpperLimitSpecify=off  RyUpperLimitBound=90  RyUpperLimitBoundUnits=deg  RyUpperLimitStiffness=1e4  RyUpperLimitStiffnessUnits=N*m/deg  RyUpperLimitDamping=10  RyUpperLimitDampingUnits=N*m/(deg/s)  RyUpperLimitTransitionRegionWidth=0.1  RyUpperLimitTransitionRegionWidthUnits=deg  RyTorqueActuationMode=NoTorque  RyMotionActuationMode=ComputedMotion  RySensePosition=off  RySenseVelocity=off  RySenseAcceleration=off  RySenseTorqueForce=off  RySenseLowerLimitTorqueForce=off  RySenseUpperLimitTorqueForce=off
  CABase : PMIOPort  Side=Right
  contact : PMIOPort  Port=2  Side=Right
  next : PMIOPort  Port=3  Side=Right
  connections:
  Arm Slice/LConn1 -- contact/RConn1
  Spring Damper 2/LConn1 -- Spring Damper 3/LConn1 -- Spring Damper 1/LConn1 -- Prismatic Joint/LConn1 -- CABase/RConn1
  Prismatic Joint/RConn1 -- Universal Joint/LConn1
  Spring Damper 1/RConn1 -- Spring Damper 2/RConn1 -- Spring Damper 3/RConn1 -- Universal Joint/RConn1 -- next/RConn1 -- Arm Slice/RConn1

== system CNN_CA_control_six_springs/Subsystem/Continuum Arm 10 ==
  Arm Slice : sm_lib/Body Elements/Cylindrical Solid  CylinderRadius=arm_radius  CylinderRadiusUnits=m  CylinderLength=arm_thickness  CylinderLengthUnits=m  ExportEntireGeometry=on  InertiaType=CalculateFromGeometry  BasedOnType=Mass  Density=1000  DensityUnits=kg/m^3  Mass=arm_mass  MassUnits=kg  CenterOfMass=[0 0 0]  CenterOfMassUnits=m  MomentsOfInertia=[1 1 1]  MomentsOfInertiaUnits=kg*m^2  ProductsOfInertia=[1 1 1]  ProductsOfInertiaUnits=kg*m^2  GraphicType=FromGeometry  MarkerShape=Sphere  MarkerSize=10  GraphicVisPropType=SimpleVisualProperties  GraphicDiffuseColor=[1.0 0 0]  GraphicOpacity=1.0  GraphicSpecularColor=[0.5 0.5 0.5 1.0]  GraphicAmbientColor=[0.15 0.15 0.15 1.0]  GraphicEmissiveColor=[0.0 0.0 0.0 1.0]  GraphicShininess=75  DoExposeReferenceFrame=on  SerializedFrames=<Frames/>
  Prismatic Joint : sm_lib/Joints/Prismatic Joint  JointMode=Normal  CompositeWrenchDir=FollowerOnBase  CompositeWrenchFrame=BaseFrame  SenseConstraintForce=off  SenseConstraintTorque=off  SenseTotalForce=off  SenseTotalTorque=off  PositionTargetSpecify=on  PositionTargetPriority=High  PositionTargetValue=ini_arm_length  PositionTargetValueUnits=m  VelocityTargetSpecify=off  VelocityTargetPriority=High  VelocityTargetValue=0  VelocityTargetValueUnits=m/s  EquilibriumPosition=0  EquilibriumPositionUnits=m  SpringStiffness=0  SpringStiffnessUnits=N/m  DampingCoefficient=0  DampingCoefficientUnits=N/(m/s)  LowerLimitSpecify=off  LowerLimitBound=-1  LowerLimitBoundUnits=m  LowerLimitStiffness=1e6  LowerLimitStiffnessUnits=N/m  LowerLimitDamping=1e3  LowerLimitDampingUnits=N/(m/s)  LowerLimitTransitionRegionWidth=1e-4  LowerLimitTransitionRegionWidthUnits=m  UpperLimitSpecify=off  UpperLimitBound=1  UpperLimitBoundUnits=m  UpperLimitStiffness=1e6  UpperLimitStiffnessUnits=N/m  UpperLimitDamping=1e3  UpperLimitDampingUnits=N/(m/s)  UpperLimitTransitionRegionWidth=1e-4  UpperLimitTransitionRegionWidthUnits=m  TorqueActuationMode=NoTorque  MotionActuationMode=ComputedMotion  SensePosition=off  SenseVelocity=off  SenseAcceleration=off  SenseTorqueForce=off  SenseLowerLimitTorqueForce=off  SenseUpperLimitTorqueForce=off
  Spring Damper 1 : Subsystem  mask{spring_position_scale=spring_position_scale_1, spring_stiffness=spring_stiffness_1, damping_coefficient=damping_coefficient_1, theta=0, row_number=1}
      mask prompts: spring_position_scale "spring position scale"; spring_stiffness "spring stiffness [N/m]"; damping_coefficient "damping coefficient [N/(m/s)]"; theta "theta [deg]"; row_number "spring label"
  Spring Damper 2 : Subsystem  mask{spring_position_scale=spring_position_scale_2, spring_stiffness=spring_stiffness_2, damping_coefficient=damping_coefficient_2, theta=120, row_number=2}
      mask prompts: spring_position_scale "spring position scale"; spring_stiffness "spring stiffness [N/m]"; damping_coefficient "damping coefficient [N/(m/s)]"; theta "theta [deg]"; row_number "spring label"
  Spring Damper 3 : Subsystem  mask{spring_position_scale=spring_position_scale_3, spring_stiffness=spring_stiffness_3, damping_coefficient=damping_coefficient_3, theta=-120, row_number=3}
      mask prompts: spring_position_scale "spring position scale"; spring_stiffness "spring stiffness [N/m]"; damping_coefficient "damping coefficient [N/(m/s)]"; theta "theta [deg]"; row_number "spring label"
  Universal Joint : sm_lib/Joints/Universal Joint  JointMode=Normal  CompositeWrenchDir=FollowerOnBase  CompositeWrenchFrame=BaseFrame  SenseConstraintForce=off  SenseConstraintTorque=off  SenseTotalForce=off  SenseTotalTorque=off  RxPositionTargetSpecify=off  RxPositionTargetPriority=High  RxPositionTargetValue=0  RxPositionTargetValueUnits=deg  RxVelocityTargetSpecify=off  RxVelocityTargetPriority=High  RxVelocityTargetValue=0  RxVelocityTargetValueUnits=deg/s  RxEquilibriumPosition=0  RxEquilibriumPositionUnits=deg  RxSpringStiffness=0  RxSpringStiffnessUnits=N*m/deg  RxDampingCoefficient=0  RxDampingCoefficientUnits=N*m/(deg/s)  RxLowerLimitSpecify=off  RxLowerLimitBound=-90  RxLowerLimitBoundUnits=deg  RxLowerLimitStiffness=1e4  RxLowerLimitStiffnessUnits=N*m/deg  RxLowerLimitDamping=10  RxLowerLimitDampingUnits=N*m/(deg/s)  RxLowerLimitTransitionRegionWidth=0.1  RxLowerLimitTransitionRegionWidthUnits=deg  RxUpperLimitSpecify=off  RxUpperLimitBound=90  RxUpperLimitBoundUnits=deg  RxUpperLimitStiffness=1e4  RxUpperLimitStiffnessUnits=N*m/deg  RxUpperLimitDamping=10  RxUpperLimitDampingUnits=N*m/(deg/s)  RxUpperLimitTransitionRegionWidth=0.1  RxUpperLimitTransitionRegionWidthUnits=deg  RxTorqueActuationMode=NoTorque  RxMotionActuationMode=ComputedMotion  RxSensePosition=off  RxSenseVelocity=off  RxSenseAcceleration=off  RxSenseTorqueForce=off  RxSenseLowerLimitTorqueForce=off  RxSenseUpperLimitTorqueForce=off  RyPositionTargetSpecify=off  RyPositionTargetPriority=High  RyPositionTargetValue=0  RyPositionTargetValueUnits=deg  RyVelocityTargetSpecify=off  RyVelocityTargetPriority=High  RyVelocityTargetValue=0  RyVelocityTargetValueUnits=deg/s  RyEquilibriumPosition=0  RyEquilibriumPositionUnits=deg  RySpringStiffness=0  RySpringStiffnessUnits=N*m/deg  RyDampingCoefficient=0  RyDampingCoefficientUnits=N*m/(deg/s)  RyLowerLimitSpecify=off  RyLowerLimitBound=-90  RyLowerLimitBoundUnits=deg  RyLowerLimitStiffness=1e4  RyLowerLimitStiffnessUnits=N*m/deg  RyLowerLimitDamping=10  RyLowerLimitDampingUnits=N*m/(deg/s)  RyLowerLimitTransitionRegionWidth=0.1  RyLowerLimitTransitionRegionWidthUnits=deg  RyUpperLimitSpecify=off  RyUpperLimitBound=90  RyUpperLimitBoundUnits=deg  RyUpperLimitStiffness=1e4  RyUpperLimitStiffnessUnits=N*m/deg  RyUpperLimitDamping=10  RyUpperLimitDampingUnits=N*m/(deg/s)  RyUpperLimitTransitionRegionWidth=0.1  RyUpperLimitTransitionRegionWidthUnits=deg  RyTorqueActuationMode=NoTorque  RyMotionActuationMode=ComputedMotion  RySensePosition=off  RySenseVelocity=off  RySenseAcceleration=off  RySenseTorqueForce=off  RySenseLowerLimitTorqueForce=off  RySenseUpperLimitTorqueForce=off
  CABase : PMIOPort  Side=Right
  contact : PMIOPort  Port=2  Side=Right
  next : PMIOPort  Port=3  Side=Right
  connections:
  Arm Slice/RConn1 -- next/RConn1 -- Universal Joint/RConn1 -- Spring Damper 3/RConn1 -- Spring Damper 2/RConn1 -- Spring Damper 1/RConn1
  Prismatic Joint/RConn1 -- Universal Joint/LConn1
  CABase/RConn1 -- Prismatic Joint/LConn1 -- Spring Damper 1/LConn1 -- Spring Damper 3/LConn1 -- Spring Damper 2/LConn1
  Arm Slice/LConn1 -- contact/RConn1
